simulink model "extremumSeekingMfcFast"  (R2015a)
settings: Solver=ode15s  StartTime=0.0  StopTime=2000  FixedStep=1e-4  RelTol=1e-9  AbsTol=1e-12
InitFcn:
  | %mfcInit = [20.8395 498.2432 2.0000 0.0412];
  | mfcInit = [5.726117682433310 0.030299840936202];
  | 
  | s0 = 300;
  | ap = 20;
  | wp = unitFreq / 10 * 2 * pi;
  | wp = 0.1;
  | wl = wp / 5;
  | wh = wl;
  | k  = 100;
  | Rinit = 1;
  | s0 = 300;
  | 
  | s0 = 600;
  | ap = 50;
  | wp = 1/60*2*pi;
  | wl = 0.26;
  | wh = .26;
  | k = 1200;
settings Model: Creator=ironi  LastModifiedBy=ironi
settings HardwareCC: ProdBitPerLong=64  ProdBitPerPointer=64  ProdWordSize=64  ProdHWDeviceType=Generic->64-bit Embedded Processor (LP64)

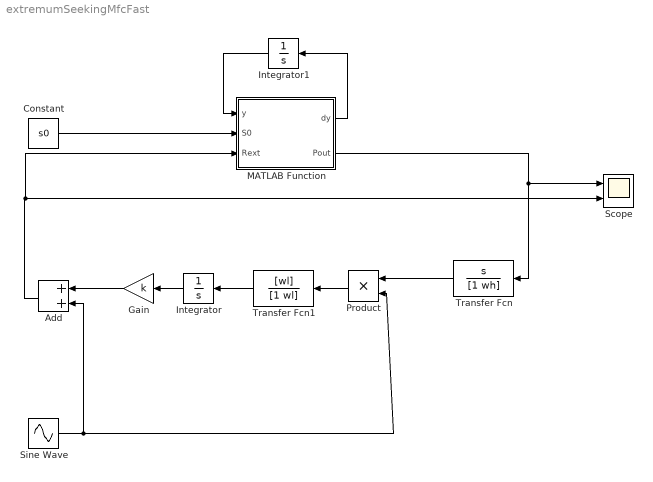
== system extremumSeekingMfcFast ==
  Add : Sum
  Constant : Constant  Value=s0
  Gain : Gain  Gain=k
  Integrator : Integrator
  Integrator1 : Integrator  InitialCondition=mfcInit
  MATLAB Function : MATLAB Function  TreatAsAtomicUnit=on
  Product : Product
  Scope : Scope  NumInputPorts=2
      settings: YMin=-5~-5  YMax=5~5
  Sine Wave : Sin  Amplitude=ap  Frequency=wp  SampleTime=0
  Transfer Fcn : TransferFcn  Numerator=[1 0]  Denominator=[1 wh]
  Transfer Fcn1 : TransferFcn  Numerator=[wl]  Denominator=[1 wl]
  wires:
  Gain/1 -> Add/1
  Integrator/1 -> Gain/1
  Transfer Fcn1/1 -> Integrator/1
  Product/1 -> Transfer Fcn1/1
  Transfer Fcn/1 -> Product/1
  Sine Wave/1 -> Add/2, Product/2
  Add/1 -> MATLAB Function/3(Rext), Scope/2
  MATLAB Function/2(Pout) -> Scope/1, Transfer Fcn/1
  Constant/1 -> MATLAB Function/2(S0)
  MATLAB Function/1(dy) -> Integrator1/1
  Integrator1/1 -> MATLAB Function/1(y)

== matlab function extremumSeekingMfcFast/MATLAB Function ==
  data: dy output; y input; S0 input; Rext input; Pout output
function [dy, Pout]= mfcModelFast(y, S0, Rext)
F = 96485;%
R = 8.314472;%
T = 298.15;%
yield = 22.753;%
% Ych4 = .3;%
qmax_a = 8.484;%
qmax_m = 8.2;%
umax_a = 1.9753;%
umax_m = .1;%
Ks_a = 20;%
Ks_m = 80;%
m = 2;%
gamma = 663400;%
Mtotal = .05;%
Km = .2*Mtotal;%
% Kd_a = .02*umax_a;%
% Kd_m = .02*umax_m;%
Xmax = 512.5;%
Kx = .01*4;%
Rmin = 25;%
Rmax = 2000 + Rmin;%
Emin = .01;%
Emax = 0.25 + 0.4144+ Emin;%
Kr = .024;%

% i0ref=0.4*4;%

e = 0.0001*Mtotal;%

V = 0.2;%
Fin = 0.1527;%

D = Fin/V;

Xtot = 500;

Xeg = 250;

S   = y(1);
Mox = y(2);
xm = Xtot - Xeg;


%% Équations dynamiques
  
Mred = Mtotal - Mox;

Rint = Rmin + (Rmax - Rmin) * exp(-Kr*Xeg);                         % (22)
Eocv = Emin + (Emax - Emin) * exp(-1/(Kr*Xeg));                     % (23)

qa = qmax_a * S / (Ks_a + S) * Mox / (Km + Mox);                    % (15)
qm = qmax_m * S / (Ks_m + S);                                       % (16)

temp = Eocv - (R*T/m/F)*abs(log(complex(Mtotal/Mred)));
Imfc = temp/(Rext+Rint)*Mred/(e+Mred);

Pout = (temp*Mred/(e+Mred)-Rint*Imfc)*Imfc;

Sp = -qa*Xeg - qm*xm + D*(S0 - S);                                   % (6)

Moxp = -yield*qa + gamma*Imfc / (m*F*V*Xeg) * 86400;                 % (12)

dy = [Sp; Moxp];
